simulink model "adaptationlaw_with_projection_op"  (R2015b)
settings: Solver=VariableStepAuto  StartTime=0.0  StopTime=10.0  RelTol=1e-3
undefined symbols (not defined in the file): b, Gamma, P, thetaEpsilon, thetaMax
settings Model: Creator=mgreiff  LastModifiedBy=mgreiff

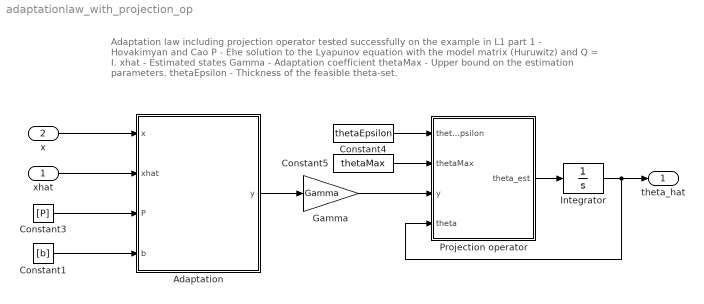
== system adaptationlaw_with_projection_op ==
  note: Adaptation law including projection operator tested successfully on the example in L1 part 1 - Hovakimyan and Cao
      |
      | P - Ehe solution to the Lyapunov equation with the model matrix (Huruwitz) and Q = I.
      | xhat - Estimated states
      | Gamma - Adaptation coefficient
      | thetaMax - Upper bound on the estimation parameters.
      | thetaEpsilon - Thickness of the feasible theta-set.
  xhat : Inport
  x : Inport  Port=2
  " Adaptation" : MATLAB Function  TreatAsAtomicUnit=on
  Constant1 : Constant  Value=[b]
  Constant3 : Constant  Value=[P]
  Constant4 : Constant  Value=thetaEpsilon
  Constant5 : Constant  Value=thetaMax
  Gamma : Gain  Gain=Gamma
  Integrator : Integrator  LimitOutput=on  UpperSaturationLimit=10  LowerSaturationLimit=-10
  Projection operator : MATLAB Function  TreatAsAtomicUnit=on
  theta_hat : Outport
  wires:
  Constant3/1 -> " Adaptation"/3(P)
  Gamma/1 -> Projection operator/3(y)
  Constant4/1 -> Projection operator/1(thetaEpsilon)
  Constant5/1 -> Projection operator/2(thetaMax)
  Projection operator/1(theta_est) -> Integrator/1
  Integrator/1 -> Projection operator/4(theta), theta_hat/1
  x/1 -> " Adaptation"/1(x)
  xhat/1 -> " Adaptation"/2(xhat)
  " Adaptation"/1(y) -> Gamma/1
  Constant1/1 -> " Adaptation"/4(b)

== matlab function adaptationlaw_with_projection_op/Projection operator ==
  data: thetaEpsilon input; thetaMax input; y input; theta_est output; theta input
function theta_est  = fcn(thetaEpsilon, thetaMax, y, theta)
%#codegen
f = (theta'*theta - thetaMax.^2)/(thetaEpsilon*thetaMax.^2);
if f < 0
    theta_est = y;
else
    nablaf = theta*2/(thetaEpsilon*thetaMax.^2);
    if nablaf'*y <= 0
        theta_est = y;
    else
        normnablaf = (nablaf/norm(nablaf));
        theta_est = y - (conj(normnablaf).*y).*normnablaf*f;
    end
end

== matlab function adaptationlaw_with_projection_op/ Adaptation ==
  data: x input; xhat input; P input; y output; b input
function y  = fcn(x, xhat, P, b)
%#codegen
xtilde = xhat-x;
y = x*xtilde'*(P*b);
